simulink model "DIesu1"  (R2020a)
settings: Solver=ode4  StartTime=0.0  StopTime=5e-4  FixedStep=1e-8  RelTol=1e-6  AbsTol=1e-6
InitFcn:
  | R1 = 1000;
  | R2 = 20;
  | L = 25.3E-6;
  | C = 100E-9;
  | IS = 1E-8;
  | UT = 26E-3;
  | f = 0.15E+6;
settings Model: Creator=LKP  LastModifiedBy=peter
settings DataIOCC: OutputOption=SpecifiedOutputTimes  OutputTimes=0:1e-8:5e-4
settings DebuggingCC: AlgebraicLoopMsg=none  ArtificialAlgebraicLoopMsg=none

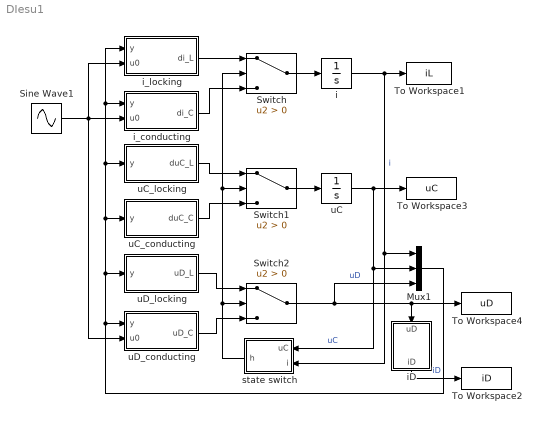
== system DIesu1 ==
  Mux1 : Mux  Inputs=3
  Sine Wave1 : Sin  Amplitude=-1  Frequency=2*pi*f  SampleTime=0
  Switch : Switch  Criteria=u2 > Threshold
  Switch1 : Switch  Criteria=u2 > Threshold
  Switch2 : Switch  Criteria=u2 > Threshold
  To Workspace1 : ToWorkspace  VariableName=iL  SaveFormat=Timeseries  SampleTime=-1
  To Workspace2 : ToWorkspace  VariableName=iD  SaveFormat=Timeseries  SampleTime=-1
  To Workspace3 : ToWorkspace  VariableName=uC  SaveFormat=Timeseries  SampleTime=-1
  To Workspace4 : ToWorkspace  VariableName=uD  SaveFormat=Timeseries  SampleTime=-1
  i : Integrator
  iD : Subsystem
      mask Display: disp('iD(uD)')
  i_conducting : Subsystem
  "i_locking " : Subsystem
  state switch : Subsystem
  uC : Integrator
  uC_conducting : Subsystem
  uC_locking : Subsystem
  uD_conducting : Subsystem
  uD_locking : Subsystem
  wires:
  uC/1 -> state switch/1(uC), Mux1/2, To Workspace3/1  "uC"
  uC_locking/1(duC_L) -> Switch1/1
  i/1 -> state switch/2(i), Mux1/1, To Workspace1/1  "i"
  Mux1/1 -> "i_locking "/1(y), i_conducting/1(y), uC_locking/1(y), uC_conducting/1(y), uD_locking/1(y), uD_conducting/1(y)
  "i_locking "/1(di_L) -> Switch/1
  i_conducting/1(di_C) -> Switch/3
  Switch/1 -> i/1
  Switch1/1 -> uC/1
  uC_conducting/1(duC_C) -> Switch1/3
  state switch/1(h) -> Switch/2, Switch1/2, Switch2/2
  uD_locking/1(uD_L) -> Switch2/1
  uD_conducting/1(uD_C) -> Switch2/3
  Switch2/1 -> Mux1/3, To Workspace4/1, iD/1(uD)  "uD"
  Sine Wave1/1 -> uD_conducting/2(u0), "i_locking "/2(u0), i_conducting/2(u0)
  iD/1(iD) -> To Workspace2/1  "iD"

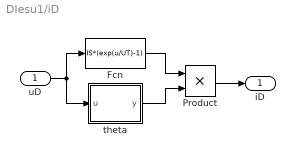
== system DIesu1/iD ==
  uD : Inport
  Fcn : Fcn  Expr=IS*(exp(u/UT)-1)
  Product : Product
  theta : Subsystem
      mask Display: text(0.5,0.5,'\fontsize{20}\Theta', 'texmode', 'on','horizontalAlignment', 'center', 'verticalAlignment', 'middle')
  iD : Outport
  wires:
  uD/1 -> theta/1(u), Fcn/1
  Fcn/1 -> Product/1
  Product/1 -> iD/1
  theta/1(y) -> Product/2

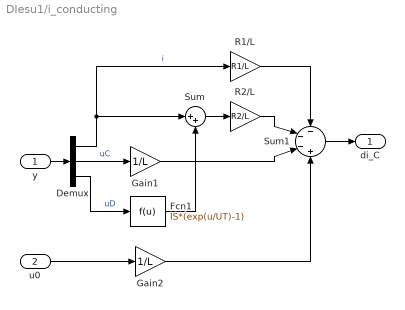
== system DIesu1/i_conducting ==
  y : Inport
  u0 : Inport  Port=2
  Demux : Demux  Outputs=3
  Fcn1 : Fcn  Expr=IS*(exp(u/UT)-1)
  Gain1 : Gain  Gain=1/L
  Gain2 : Gain  Gain=1/L
  R1/L : Gain  Gain=R1/L
  R2/L : Gain  Gain=R2/L
  Sum : Sum  Inputs=|++
  Sum1 : Sum  Inputs=---+
  di_C : Outport
  wires:
  y/1 -> Demux/1
  Demux/1 -> R1/L/1, Sum/1  "i"
  Demux/3 -> Fcn1/1  "uD"
  Fcn1/1 -> Sum/2
  Sum/1 -> R2/L/1
  Demux/2 -> Gain1/1  "uC"
  R1/L/1 -> Sum1/1
  R2/L/1 -> Sum1/2
  Gain1/1 -> Sum1/3
  Sum1/1 -> di_C/1
  u0/1 -> Gain2/1
  Gain2/1 -> Sum1/4

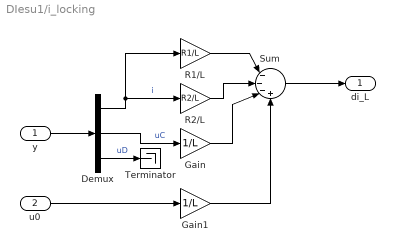
== system DIesu1/i_locking  ==
  y : Inport
  u0 : Inport  Port=2
  Demux : Demux  Outputs=3
  Gain : Gain  Gain=1/L
  Gain1 : Gain  Gain=1/L
  R1/L : Gain  Gain=R1/L
  R2/L : Gain  Gain=R2/L
  Sum : Sum  Inputs=|---+
  Terminator : Terminator
  di_L : Outport
  wires:
  y/1 -> Demux/1
  Demux/2 -> Gain/1  "uC"
  Sum/1 -> di_L/1
  R1/L/1 -> Sum/1
  Demux/1 -> R2/L/1, R1/L/1  "i"
  R2/L/1 -> Sum/2
  Gain/1 -> Sum/3
  Gain1/1 -> Sum/4
  Demux/3 -> Terminator/1  "uD"
  u0/1 -> Gain1/1

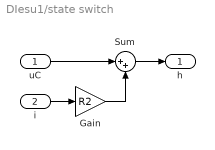
== system DIesu1/state switch ==
  uC : Inport
  i : Inport  Port=2
  Gain : Gain  Gain=R2
  Sum : Sum  Inputs=|++
  h : Outport
  wires:
  uC/1 -> Sum/1
  Sum/1 -> h/1
  i/1 -> Gain/1
  Gain/1 -> Sum/2

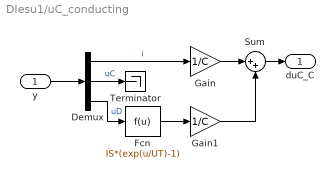
== system DIesu1/uC_conducting ==
  y : Inport
  Demux : Demux  Outputs=3
  Fcn : Fcn  Expr=IS*(exp(u/UT)-1)
  Gain : Gain  Gain=1/C
  Gain1 : Gain  Gain=1/C
  Sum : Sum  Inputs=|++
  Terminator : Terminator
  duC_C : Outport
  wires:
  Gain/1 -> Sum/1
  Sum/1 -> duC_C/1
  y/1 -> Demux/1
  Demux/1 -> Gain/1  "i"
  Demux/2 -> Terminator/1  "uC"
  Demux/3 -> Fcn/1  "uD"
  Fcn/1 -> Gain1/1
  Gain1/1 -> Sum/2

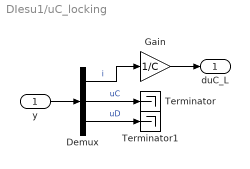
== system DIesu1/uC_locking ==
  y : Inport
  Demux : Demux  Outputs=3
  Gain : Gain  Gain=1/C
  Terminator : Terminator
  Terminator1 : Terminator
  duC_L : Outport
  wires:
  y/1 -> Demux/1
  Demux/1 -> Gain/1  "i"
  Gain/1 -> duC_L/1
  Demux/2 -> Terminator/1  "uC"
  Demux/3 -> Terminator1/1  "uD"

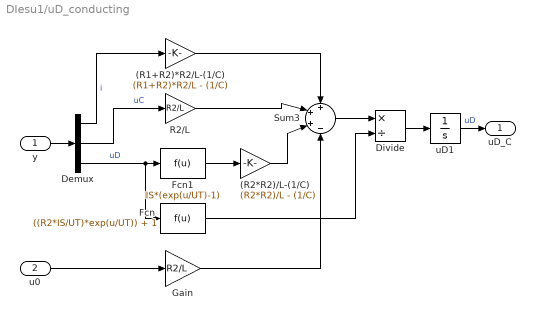
== system DIesu1/uD_conducting ==
  y : Inport
  u0 : Inport  Port=2
  (R1+R2)*R2/L-(1/C) : Gain  Gain=(R1+R2)*R2/L - (1/C)
  (R2*R2)/L-(1/C) : Gain  Gain=(R2*R2)/L - (1/C)
  Demux : Demux  Outputs=3
  Divide : Product  Inputs=*/
  Fcn : Fcn  Expr=((R2*IS/UT)*exp(u/UT)) + 1
  Fcn1 : Fcn  Expr=IS*(exp(u/UT)-1)
  Gain : Gain  Gain=R2/L
  R2/L : Gain  Gain=R2/L
  Sum3 : Sum  Inputs=+++-
  uD1 : Integrator
  uD_C : Outport
  wires:
  y/1 -> Demux/1
  (R2*R2)/L-(1/C)/1 -> Sum3/3
  Fcn/1 -> Divide/2
  (R1+R2)*R2/L-(1/C)/1 -> Sum3/1
  u0/1 -> Gain/1
  R2/L/1 -> Sum3/2
  Fcn1/1 -> (R2*R2)/L-(1/C)/1
  Gain/1 -> Sum3/4
  Sum3/1 -> Divide/1
  Demux/2 -> R2/L/1  "uC"
  Demux/1 -> (R1+R2)*R2/L-(1/C)/1  "i"
  Demux/3 -> Fcn/1, Fcn1/1  "uD"
  Divide/1 -> uD1/1
  uD1/1 -> uD_C/1  "uD"

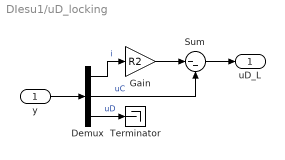
== system DIesu1/uD_locking ==
  y : Inport
  Demux : Demux  Outputs=3
  Gain : Gain  Gain=R2
  Sum : Sum  Inputs=|--
  Terminator : Terminator
  uD_L : Outport
  wires:
  Demux/1 -> Gain/1  "i"
  Gain/1 -> Sum/1
  Demux/2 -> Sum/2  "uC"
  Demux/3 -> Terminator/1  "uD"
  y/1 -> Demux/1
  Sum/1 -> uD_L/1

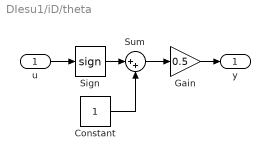
== system DIesu1/iD/theta ==
  u : Inport
  Constant : Constant
  Gain : Gain  Gain=0.5
  Sign : Signum
  Sum : Sum  Inputs=|++
  y : Outport
  wires:
  Sum/1 -> Gain/1
  u/1 -> Sign/1
  Constant/1 -> Sum/2
  Sign/1 -> Sum/1
  Gain/1 -> y/1
